simulink library "HEV_Electrical_Lib"  (R2024b)
settings: Solver=ode23t  StartTime=0.0  StopTime=10  MaxStep=1e-3  RelTol=1e-3
values from neighbouring files (symbols this model uses):
  Ts = 2e-6    (= 2e-06)    [param.m]
undefined symbols (not defined in the file or in its folder): DiscIntNeverNeededParam, HEV_Param, magnitude
libraries: fl_lib x73, nesl_utility x30, spsCurrentMeasurementLib x23, spsIdealSwitchLib x12, spsVoltageMeasurementLib x11, simulink_extras x8, spsControlledCurrentSourceLib x7, spsSeriesRLCBranchLib x6, simulink x6, spsControlledVoltageSourceLib x5, spsPermanentMagnetSynchronousMachineLib x4, spsUniversalBridgeLib x3
(part 4 of 4)

== system HEV_Electrical_Lib/Subsystem/System Level/DC-DC Converter/Thermal Model ==
  Air Temperature : fl_lib/Physical Signals/Sources/PS Constant  constant=HEV_Param.DCDCConv.Air_Temperature
  Ideal Heat Flow Source : fl_lib/Thermal/Thermal Sources/Controlled Heat Flow Rate Source
  Ideal Temperature Source : fl_lib/Thermal/Thermal Sources/Controlled Temperature Source
  Nominal Case-Atmosphere Convective Heat Transfer : fl_lib/Thermal/Thermal Elements/Convective Heat Transfer  thermal_type=foundation.enum.constant_variable.constant  area=HEV_Param.DCDCConv.Convection.Area cm^2  heat_tr_coeff=HEV_Param.DCDCConv.Convection.HT_Coefficient W/(m^2 *K)  min_heat_tr_coeff=1e-3 W/(K*m^2)  T_specify=off  T_priority=High  T=0 K  T_nominal_specify=off  T_nominal_value=1  T_nominal_unit=K  Q_specify=off  Q_priority=High  Q=0 J/s  Q_nominal_specify=off  Q_nominal_value=1  Q_nominal_unit=J/s
  PtoHeat : fl_lib/Physical Signals/Functions/PS Gain  gain=HEV_Param.DCDCConv.EPower2Heat
  Subsystem : Subsystem
      mask Display: disp('S');
  Temperature Sensor : Subsystem
      mask Display:
      | patch([294.730220921338;294.546109275896;293.995547435362;293.083837611228;291.819760067491;290.215488561913;288.286473106077;286.051291173329;283.531468787557;280.75127321581;277.737479261253;274.519111407178;271.127164295357;267.594304230703;263.954554586898;260.242968142701;256.495289504528;252.747610866356;249.036024422158;245.396274778353;241.8634147137;238.471467601878;235.253099747803;232.239305793246;229.459110221499;226.939287835727;224.704105902979;222.775090447143;221.170818941565;219.906741397828;218.995031573694;218.44446973316;218.260358087718;218.44446973316;218.995031573694;219.906741397828;221.170818941565;222.775090447143;224.704105902979;226.939287835727;229.459110221499;232.239305793247;235.253099747803;238.471467601878;241.8634147137;245.396274778353;249.036024422158;252.747610866356;256.495289504528;260.242968142701;263.954554586898;267.594304230703;271.127164295357;274.519111407178;277.737479261253;280.75127321581;283.531468787557;286.051291173329;288.286473106077;290.215488561913;291.819760067491;293.083837611228;293.995547435362;294.546109275896;294.730220921338;294.730220921338], [122.389574535191;118.641895897019;114.930309452821;111.290559809016;107.757699744363;104.365752632541;101.147384778466;98.1335908239095;95.3533952521624;92.8335728663899;90.598390933642;88.6693754778057;87.0651039722279;85.8010264284914;84.8893166043572;84.3387547638233;84.1546431183815;84.3387547638233;84.8893166043572;85.8010264284914;87.0651039722279;88.6693754778058;90.598390933642;92.83357286639;95.3533952521625;98.1335908239095;101.147384778466;104.365752632541;107.757699744363;111.290559809016;114.930309452821;118.641895897019;122.389574535191;126.137253173364;129.848839617561;133.488589261366;137.02144932602;140.413396437841;143.631764291917;146.645558246473;149.42575381822;151.945576203992;154.18075813674;156.109773592576;157.714045098154;158.978122641891;159.889832466025;160.440394306559;160.624505952001;160.440394306559;159.889832466025;158.978122641891;157.714045098154;156.109773592576;154.18075813674;151.945576203992;149.42575381822;146.645558246473;143.631764291917;140.413396437841;137.02144932602;133.488589261366;129.848839617561;126.137253173364;122.389574535191;122.389574535191], [0;0;0])
      | plot([294.730220921338;294.546109275896;293.995547435362;293.083837611228;291.819760067491;290.215488561913;288.286473106077;286.051291173329;283.531468787557;280.75127321581;277.737479261253;274.519111407178;271.127164295357;267.594304230703;263.954554586898;260.242968142701;256.495289504528;252.747610866356;249.036024422158;245.396274778353;241.8634147137;238.471467601878;235.253099747803;232.239305793246;229.459110221499;226.939287835727;224.704105902979;222.775090447143;221.170818941565;219.906741397828;218.995031573694;218.44446973316;218.260358087718;218.44446973316;218.995031573694;219.906741397828;221.170818941565;222.775090447143;224.704105902979;226.939287835727;229.459110221499;232.239305793247;235.253099747803;238.471467601878;241.8634147137;245.396274778353;249.036024422158;252.747610866356;256.495289504528;260.242968142701;263.954554586898;267.594304230703;271.127164295357;274.519111407178;277.737479261253;280.75127321581;283.531468787557;286.051291173329;288.286473106077;290.215488561913;291.819760067491;293.083837611228;293.995547435362;294.546109275896;294.730220921338;294.730220921338], [122.389574535191;118.641895897019;114.930309452821;111.290559809016;107.757699744363;104.365752632541;101.147384778466;98.1335908239095;95.3533952521624;92.8335728663899;90.598390933642;88.6693754778057;87.0651039722279;85.8010264284914;84.8893166043572;84.3387547638233;84.1546431183815;84.3387547638233;84.8893166043572;85.8010264284914;87.0651039722279;88.6693754778058;90.598390933642;92.83357286639;95.3533952521625;98.1335908239095;101.147384778466;104.365752632541;107.757699744363;111.290559809016;114.930309452821;118.641895897019;122.389574535191;126.137253173364;129.848839617561;133.488589261366;137.02144932602;140.413396437841;143.631764291917;146.645558246473;149.42575381822;151.945576203992;154.18075813674;156.109773592576;157.714045098154;158.978122641891;159.889832466025;160.440394306559;160.624505952001;160.440394306559;159.889832466025;158.978122641891;157.714045098154;156.109773592576;154.18075813674;151.945576203992;149.42575381822;146.645558246473;143.631764291917;140.413396437841;137.02144932602;133.488589261366;129.848839617561;126.137253173364;122.389574535191;122.389574535191])
      | plot([243.771309033036;263.613159768283;263.613159768283;243.771309033036;243.771309033036], [438.410416245461;438.410416245461;112.4371541664;112.4371541664;438.410416245461])
      | plot([510.219018906355;0;0;510.219018906355;510.219018906355], [509.274168871343;509.274168871343;0;0;509.274168871343])
      | ;
      | %color('red');
      | %port_label('LConn', 1,'A')
      | %port_label('RConn', 1,'B')
  Thermal Mass : fl_lib/Thermal/Thermal Elements/Thermal Mass  mass_type=foundation.enum.constant_variable.constant  mass=HEV_Param.DCDCConv.Thermal_Mass kg  sp_heat=HEV_Param.DCDCConv.Specific_Heat J/kg/K  mass_min=1e-6 kg  num_ports=foundation.enum.numPorts2.one  m_specify=off  m_priority=High  m=1 kg  m_nominal_specify=off  m_nominal_value=1  m_nominal_unit=kg  T_specify=on  T_priority=High  T=HEV_Param.DCDCConv.Initial_Temperature degC  T_nominal_specify=off  T_nominal_value=1  T_nominal_unit=K  Q_specify=off  Q_priority=High  Q=0 J/s  Q_nominal_specify=off  Q_nominal_value=1  Q_nominal_unit=J/s
  Thermal Reference : fl_lib/Thermal/Thermal Elements/Thermal Reference
  Thermal Reference1 : fl_lib/Thermal/Thermal Elements/Thermal Reference
  P Loss : PMIOPort  Side=Left
  connections:
  Nominal Case-Atmosphere Convective Heat Transfer/LConn1 -- Ideal Temperature Source/LConn1
  Temperature Sensor/LConn1 -- Nominal Case-Atmosphere Convective Heat Transfer/RConn1 -- Thermal Mass/LConn1 -- Ideal Heat Flow Source/LConn1
  PtoHeat/RConn1 -- Ideal Heat Flow Source/RConn1
  Ideal Temperature Source/RConn2 -- Thermal Reference/LConn1
  Air Temperature/RConn1 -- Ideal Temperature Source/RConn1
  Subsystem/LConn1 -- P Loss/RConn1
  PtoHeat/LConn1 -- Subsystem/RConn1
  Thermal Reference1/LConn1 -- Ideal Heat Flow Source/RConn2

== system HEV_Electrical_Lib/Subsystem/System Level/DC-DC Converter/Voltage Sensor ==
  PS-Simulink Converter : nesl_utility/PS-Simulink Converter  PhysicalDomain=network_engine_domain  SubClassName=ps_output  LeftPortType=input  RightPortType=output  PseudoPeriodic=off  Frequencies=[]  VectorFormat=1-D array  Unit=1  AffineConversion=off
  Voltage Sensor In : fl_lib/Electrical/Electrical Sensors/Voltage Sensor
  + : PMIOPort  Side=Left
  V : PMIOPort  Port=2  Side=Right
  - : PMIOPort  Port=3  Side=Right
  tag scope: V_in=global
  wires:
  PS-Simulink Converter/1 -> [V_in]
  connections:
  +/RConn1 -- Voltage Sensor In/LConn1
  -/RConn1 -- Voltage Sensor In/RConn2
  V/RConn1 -- Voltage Sensor In/RConn1 -- PS-Simulink Converter/LConn1

== system HEV_Electrical_Lib/Subsystem/System Level/DC-DC Converter/Voltage Sensor Bus ==
  PS-Simulink Converter : nesl_utility/PS-Simulink Converter  PhysicalDomain=network_engine_domain  SubClassName=ps_output  LeftPortType=input  RightPortType=output  PseudoPeriodic=off  Frequencies=[]  VectorFormat=1-D array  Unit=1  AffineConversion=off
  Voltage Sensor Out : fl_lib/Electrical/Electrical Sensors/Voltage Sensor
  + : PMIOPort  Side=Left
  - : PMIOPort  Port=2  Side=Right
  V : PMIOPort  Port=3  Side=Right
  tag scope: V_out=global
  wires:
  PS-Simulink Converter/1 -> [V_out]
  connections:
  +/RConn1 -- Voltage Sensor Out/LConn1
  V/RConn1 -- Voltage Sensor Out/RConn1 -- PS-Simulink Converter/LConn1
  -/RConn1 -- Voltage Sensor Out/RConn2

== system HEV_Electrical_Lib/Subsystem/System Level/Synchronous Motor & Drive/GF ==
  In1 : Inport
  Simulink-PS Converter : nesl_utility/Simulink-PS Converter  PhysicalDomain=network_engine_domain  SubClassName=ps_input  LeftPortType=input  RightPortType=output  PseudoPeriodic=off  Frequencies=[]  NoiseDistribution=none  NoiseParameters=[]  Unit=1  AffineConversion=off  FilteringAndDerivatives=zero  SimscapeFilterOrder=1  InputFilterTimeConstant=0.005  UdotUserProvided=0
  Conn1 : PMIOPort  Side=Right
  tag scope: Mot_TReq_SYS=global
  wires:
  In1/1 -> [Mot_TReq_SYS], Simulink-PS Converter/1
  connections:
  Simulink-PS Converter/RConn1 -- Conn1/RConn1

== system HEV_Electrical_Lib/Subsystem/System Level/Synchronous Motor & Drive/PS Terminator1 ==
  PS-Simulink Converter 2 : nesl_utility/PS-Simulink Converter  PhysicalDomain=network_engine_domain  SubClassName=ps_output  LeftPortType=input  RightPortType=output  PseudoPeriodic=off  Frequencies=[]  VectorFormat=1-D array  Unit=rpm  AffineConversion=off
  Terminator : Terminator
  R : PMIOPort  Side=Left
  wires:
  PS-Simulink Converter 2/1 -> Terminator/1
  connections:
  R/RConn1 -- PS-Simulink Converter 2/LConn1

== system HEV_Electrical_Lib/Subsystem/System Level/Synchronous Motor & Drive/Power Sensor ==
  Current Sensor : fl_lib/Electrical/Electrical Sensors/Current Sensor
  PS Product1 : fl_lib/Physical Signals/Functions/PS Product
  PS-Simulink Converter4 : nesl_utility/PS-Simulink Converter  PhysicalDomain=network_engine_domain  SubClassName=ps_output  LeftPortType=input  RightPortType=output  PseudoPeriodic=off  Frequencies=[]  VectorFormat=1-D array  Unit=W  AffineConversion=off
  Voltage Sensor : fl_lib/Electrical/Electrical Sensors/Voltage Sensor
  W to kW : Gain  Gain=1/1000
  + : PMIOPort  Side=Left
  ref : PMIOPort  Port=2  Side=Left
  - : PMIOPort  Port=3  Side=Right
  tag scope: Pe_motor=global
  wires:
  W to kW/1 -> [Pe_motor]
  PS-Simulink Converter4/1 -> W to kW/1
  connections:
  Current Sensor/RConn1 -- PS Product1/LConn1
  -/RConn1 -- Current Sensor/RConn2 -- Voltage Sensor/LConn1
  Voltage Sensor/RConn1 -- PS Product1/LConn2
  PS-Simulink Converter4/LConn1 -- PS Product1/RConn1
  +/RConn1 -- Current Sensor/LConn1
  ref/RConn1 -- Voltage Sensor/RConn2

== system HEV_Electrical_Lib/Subsystem/System Level/Synchronous Motor & Drive/Power and Torque Sensor ==
  Ideal Rotational Motion Sensor : fl_lib/Mechanical/Mechanical Sensors/Ideal Rotational Motion Sensor  reference=foundation.enum.MeasurementReference.difference  acceleration_port=false  velocity_port=true  position_port=true  wrap_angle=simscape.enum.onoff.off  offset=0 rad
  Mechanical Rotational Reference1 : fl_lib/Mechanical/Rotational Elements/Mechanical Rotational Reference
  PS Product : fl_lib/Physical Signals/Functions/PS Product
  PS-Simulink Converter3 : nesl_utility/PS-Simulink Converter  PhysicalDomain=network_engine_domain  SubClassName=ps_output  LeftPortType=input  RightPortType=output  PseudoPeriodic=off  Frequencies=[]  VectorFormat=1-D array  Unit=W  AffineConversion=off
  Torque Sensor : fl_lib/Mechanical/Mechanical Sensors/Ideal Torque Sensor
  W to kW : Gain  Gain=1/1000
  C : PMIOPort  Side=Right
  R : PMIOPort  Port=2  Side=Left
  tag scope: Pm_motor=global
  wires:
  PS-Simulink Converter3/1 -> W to kW/1
  W to kW/1 -> [Pm_motor]
  connections:
  C/RConn1 -- Torque Sensor/RConn1
  R/RConn1 -- Torque Sensor/LConn1 -- Ideal Rotational Motion Sensor/LConn1
  PS Product/RConn1 -- PS-Simulink Converter3/LConn1
  Torque Sensor/RConn2 -- PS Product/LConn1
  Ideal Rotational Motion Sensor/RConn2 -- PS Product/LConn2
  Mechanical Rotational Reference1/LConn1 -- Ideal Rotational Motion Sensor/RConn1

== system HEV_Electrical_Lib/Detailed/DC//DC Converter/PWM/Thermal Model/Subsystem ==
  IBus : Inport
  PToHeat : Gain  Gain=HEV_Param.DCDCConv.EPower2Heat  SaturateOnIntegerOverflow=on  OutDataTypeStr=Inherit: Same as input  ParamDataTypeStr=Inherit: Same as input
  Product : Product  RndMeth=Zero
  RLoss : Gain  Gain=HEV_Param.DCDCConv.Resistance_Losses  SaturateOnIntegerOverflow=on  OutDataTypeStr=Inherit: Same as input  ParamDataTypeStr=Inherit: Same as input
  Heat Flow : Outport  VectorParamsAs1DForOutWhenUnconnected=off
  wires:
  Product/1 -> RLoss/1
  IBus/1 -> Product/1, Product/2
  RLoss/1 -> PToHeat/1
  PToHeat/1 -> Heat Flow/1

== system HEV_Electrical_Lib/Mean Value/DC//DC Converter/Boost Converter Average-Values/Thermal Model/Subsystem ==
  IBus : Inport
  PToHeat : Gain  Gain=HEV_Param.DCDCConv.EPower2Heat  SaturateOnIntegerOverflow=on  OutDataTypeStr=Inherit: Same as input  ParamDataTypeStr=Inherit: Same as input
  Product : Product  RndMeth=Zero
  RLoss : Gain  Gain=HEV_Param.DCDCConv.Resistance_Losses  SaturateOnIntegerOverflow=on  OutDataTypeStr=Inherit: Same as input  ParamDataTypeStr=Inherit: Same as input
  Heat Flow : Outport  VectorParamsAs1DForOutWhenUnconnected=off
  wires:
  PToHeat/1 -> Heat Flow/1
  RLoss/1 -> PToHeat/1
  IBus/1 -> Product/2, Product/1
  Product/1 -> RLoss/1

== system HEV_Electrical_Lib/Mean Value/Synchronous Generator & Drive/Three-phase Inverter/Id computation/Demux ==
  m : Inport
  Demux1 : Demux  Outputs=5
      settings: DisplayOption=none
  Terminator : Terminator
  Vac : Outport  VectorParamsAs1DForOutWhenUnconnected=off
  Ia : Outport  Port=2  VectorParamsAs1DForOutWhenUnconnected=off
  Vbc : Outport  Port=3  VectorParamsAs1DForOutWhenUnconnected=off
  Ib : Outport  Port=4  VectorParamsAs1DForOutWhenUnconnected=off
  wires:
  m/1 -> Demux1/1
  Demux1/5 -> Vbc/1  "Vbc"
  Demux1/4 -> Vac/1  "Vac"
  Demux1/2 -> Ib/1  "Ib"
  Demux1/1 -> Ia/1  "Ia"
  Demux1/3 -> Terminator/1  "Ic"

== system HEV_Electrical_Lib/Mean Value/Synchronous Generator & Drive/Three-phase Inverter/Id computation/Demux1 ==
  m : Inport
  Demux1 : Demux  Outputs=5
      settings: DisplayOption=none
  Terminator1 : Terminator
  Terminator2 : Terminator
  Ia : Outport  VectorParamsAs1DForOutWhenUnconnected=off
  Ib : Outport  Port=2  VectorParamsAs1DForOutWhenUnconnected=off
  Ic : Outport  Port=3  VectorParamsAs1DForOutWhenUnconnected=off
  wires:
  Demux1/3 -> Ic/1  "Ic"
  Demux1/1 -> Ia/1  "Ia"
  Demux1/2 -> Ib/1  "Ib"
  Demux1/4 -> Terminator1/1  "Vac"
  Demux1/5 -> Terminator2/1  "Vbc"
  m/1 -> Demux1/1

== system HEV_Electrical_Lib/Mean Value/Synchronous Motor & Drive/Three-phase Inverter/Id computation/Demux ==
  m : Inport
  Demux1 : Demux  Outputs=5
      settings: DisplayOption=none
  Terminator : Terminator
  Vac : Outport  VectorParamsAs1DForOutWhenUnconnected=off
  Ia : Outport  Port=2  VectorParamsAs1DForOutWhenUnconnected=off
  Vbc : Outport  Port=3  VectorParamsAs1DForOutWhenUnconnected=off
  Ib : Outport  Port=4  VectorParamsAs1DForOutWhenUnconnected=off
  wires:
  Demux1/3 -> Terminator/1  "Ic"
  Demux1/1 -> Ia/1  "Ia"
  Demux1/2 -> Ib/1  "Ib"
  Demux1/4 -> Vac/1  "Vac"
  Demux1/5 -> Vbc/1  "Vbc"
  m/1 -> Demux1/1

== system HEV_Electrical_Lib/Mean Value/Synchronous Motor & Drive/Three-phase Inverter/Id computation/Demux1 ==
  m : Inport
  Demux1 : Demux  Outputs=5
      settings: DisplayOption=none
  Terminator1 : Terminator
  Terminator2 : Terminator
  Ia : Outport  VectorParamsAs1DForOutWhenUnconnected=off
  Ib : Outport  Port=2  VectorParamsAs1DForOutWhenUnconnected=off
  Ic : Outport  Port=3  VectorParamsAs1DForOutWhenUnconnected=off
  wires:
  m/1 -> Demux1/1
  Demux1/5 -> Terminator2/1  "Vbc"
  Demux1/4 -> Terminator1/1  "Vac"
  Demux1/2 -> Ib/1  "Ib"
  Demux1/1 -> Ia/1  "Ia"
  Demux1/3 -> Ic/1  "Ic"

== system HEV_Electrical_Lib/Subsystem/System Level/DC-DC Converter/Thermal Model/Subsystem ==
  PS-Simulink Converter1 : nesl_utility/PS-Simulink Converter  PhysicalDomain=network_engine_domain  SubClassName=ps_output  LeftPortType=input  RightPortType=output  PseudoPeriodic=off  Frequencies=[]  VectorFormat=1-D array  Unit=W  AffineConversion=on
  In : PMIOPort  Side=Left
  Out : PMIOPort  Port=2  Side=Right
  tag scope: DCDC_Power_Loss=global
  wires:
  PS-Simulink Converter1/1 -> [DCDC_Power_Loss]
  connections:
  In/RConn1 -- PS-Simulink Converter1/LConn1 -- Out/RConn1

== system HEV_Electrical_Lib/Subsystem/System Level/DC-DC Converter/Thermal Model/Temperature Sensor ==
  Ideal Temperature Sensor : fl_lib/Thermal/Thermal Sensors/Temperature Sensor  temperature_measure=foundation.enum.MeasurementReference.difference
  PS-Simulink Converter : nesl_utility/PS-Simulink Converter  PhysicalDomain=network_engine_domain  SubClassName=ps_output  LeftPortType=input  RightPortType=output  PseudoPeriodic=off  Frequencies=[]  VectorFormat=1-D array  Unit=degC  AffineConversion=on
  Thermal Reference : fl_lib/Thermal/Thermal Elements/Thermal Reference
  Conn2 : PMIOPort  Side=Left
  tag scope: DCDC_SYS=global
  wires:
  PS-Simulink Converter/1 -> [DCDC_SYS]  "DCDC_Temp"
  connections:
  PS-Simulink Converter/LConn1 -- Ideal Temperature Sensor/RConn2
  Thermal Reference/LConn1 -- Ideal Temperature Sensor/RConn1
  Conn2/RConn1 -- Ideal Temperature Sensor/LConn1

== matlab function HEV_Electrical_Lib/Mean Value/Synchronous Motor & Drive/VECT controller/Embedded MATLAB Function1 ==
  data: iqn_opt input; Ten input; iqn output; w input; Vdc input; params input; idn output
function [iqn,idn] = fcn(iqn_opt,Ten,w,Vdc,params)
% This block supports the Embedded MATLAB subset.
% See the help menu for details.

kFact = 0.9;
Ld = params(1);
Lq = params(2);
lam = params(3);
p = params(4);
ib = params(5);
Vs = Vdc/(pi/2)*kFact;
ten = abs(Ten);
iqn = sign(Ten)*iqn_opt;
if Ten == 0 && w == 0
    idn = 0;
elseif iqn == 0
    idn = -(lam*p*w-Vs*kFact)/(p*Ld*w*ib);
else
    idn = 1-Ten/iqn;
end
if sqrt((-Lq*p*w*iqn*ib)^2+(Ld*p*w*idn*ib+lam*p*w)^2) >= Vs 
    vs = Vs;
    k1 = 2*lam*Ld/(ib*Lq^2);
    k2 = Ld^2/Lq^2;
    k3 = lam^2/(ib^2*Lq^2)+k2;
    
    g2 = -vs^2/(p^2*ib^2*Lq^2*w^2) + k1 + k3;
    g3 = -k1*ten-2*ten*k2;
    g4 = k2*ten^2;
    
    a1 = abs(-768*g4^3+384*g4^2*g2^2-48*g4*g2^4-432*g2*g4*g3^2+81*g3^4+12*g3^2*g2^3)^(1/2);
    a2 = (-288*g2*g4+108*g3^2+8*g2^3+12*a1)^(1/3);
    a3 = (-4*g2+a2+48/a2*g4+4/a2*g2^2)^(1/2);
    iqn = (1/12*6^(1/2)*a3+1/12*abs(-48*g2-6*a2-288/a2*g4-24/a2*g2^2-72/a3*g3*6^(1/2))^(1/2));
    iqn = sign(Ten)*iqn;

    idn = 1-Ten/iqn;
end

== matlab function HEV_Electrical_Lib/Detailed/Synchronous Motor & Drive/VECT Controller/Embedded MATLAB Function1 ==
  data: iqn_opt input; Ten input; iqn output; w input; Vdc input; params input; idn output
function [iqn,idn] = fcn(iqn_opt,Ten,w,Vdc,params)
% This block supports the Embedded MATLAB subset.
% See the help menu for details.

kFact = 0.9;
Ld = params(1);
Lq = params(2);
lam = params(3);
p = params(4);
ib = params(5);
Vs = Vdc/(pi/2)*kFact;
ten = abs(Ten);
iqn = sign(Ten)*iqn_opt;
if Ten == 0 && w == 0
    idn = 0;
elseif iqn == 0
    idn = -(lam*p*w-Vs*kFact)/(p*Ld*w*ib);
else
    idn = 1-Ten/iqn;
end
if sqrt((-Lq*p*w*iqn*ib)^2+(Ld*p*w*idn*ib+lam*p*w)^2) >= Vs 
    vs = Vs;
    k1 = 2*lam*Ld/(ib*Lq^2);
    k2 = Ld^2/Lq^2;
    k3 = lam^2/(ib^2*Lq^2)+k2;
    
    g2 = -vs^2/(p^2*ib^2*Lq^2*w^2) + k1 + k3;
    g3 = -k1*ten-2*ten*k2;
    g4 = k2*ten^2;
    
    a1 = abs(-768*g4^3+384*g4^2*g2^2-48*g4*g2^4-432*g2*g4*g3^2+81*g3^4+12*g3^2*g2^3)^(1/2);
    a2 = (-288*g2*g4+108*g3^2+8*g2^3+12*a1)^(1/3);
    a3 = (-4*g2+a2+48/a2*g4+4/a2*g2^2)^(1/2);
    iqn = (1/12*6^(1/2)*a3+1/12*abs(-48*g2-6*a2-288/a2*g4-24/a2*g2^2-72/a3*g3*6^(1/2))^(1/2));
    iqn = sign(Ten)*iqn;

    idn = 1-Ten/iqn;
end
